simulink library "misc_modbus_genbatt_lib"  (Simulink 8.1)
settings: Solver=ode45  StartTime=0.0  StopTime=10.0  RelTol=1e-3
libraries: rtio_generic_modbus x3, simulink x1
settings Model: Creator=RE25624  LastModifiedBy=RE25624

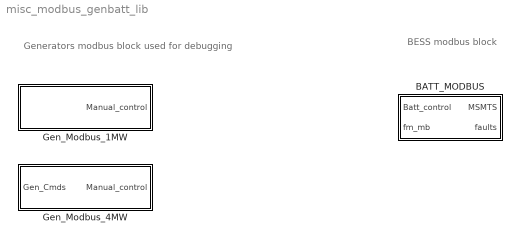
== system misc_modbus_genbatt_lib ==
  note: BESS modbus block
  note: Generators modbus block used for debugging
  BATT_MODBUS : Subsystem
  Gen_Modbus_1MW : Subsystem
  Gen_Modbus_4MW : Subsystem

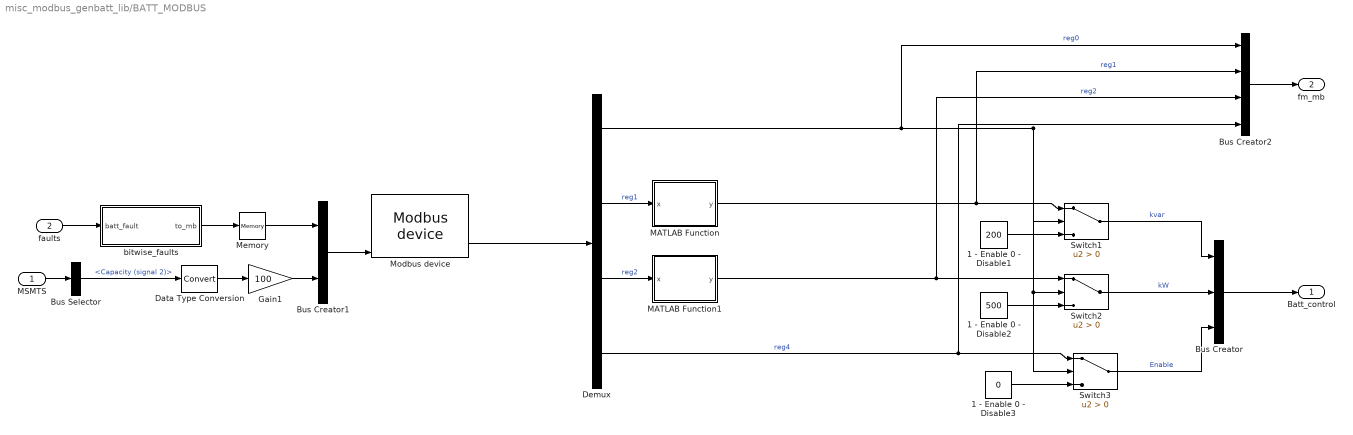
== system misc_modbus_genbatt_lib/BATT_MODBUS ==
  MSMTS : Inport
  faults : Inport  Port=2
  1 - Enable 0 - Disable1 : Constant  Value=200
  1 - Enable 0 - Disable2 : Constant  Value=500
  1 - Enable 0 - Disable3 : Constant  Value=0
  Bus Creator : BusCreator  Inputs=3
  Bus Creator1 : BusCreator  Inputs=2
  Bus Creator2 : BusCreator
  Bus Selector : BusSelector  OutputSignals=Capacity (signal 2)
  Data Type Conversion : DataTypeConversion
  Demux : Demux
  Gain1 : Gain  Gain=100
  MATLAB Function : MATLAB Function  TreatAsAtomicUnit=on
  MATLAB Function1 : MATLAB Function  TreatAsAtomicUnit=on
  Memory : Memory
  Modbus device : rtio_generic_modbus/Modbus device  conf_name=batt_slave_cfg.opal  conf_name_mask=batt_slave_cfg.xls  sample_time=Ts
  Switch1 : Switch  Criteria=u2 > Threshold
  Switch2 : Switch  Criteria=u2 > Threshold
  Switch3 : Switch  Criteria=u2 > Threshold
  bitwise_faults : Subsystem
  Batt_control : Outport
  fm_mb : Outport  Port=2
  wires:
  Modbus device/2 -> Demux/1
  1 - Enable 0 - Disable1/1 -> Switch1/3
  1 - Enable 0 - Disable2/1 -> Switch2/3
  1 - Enable 0 - Disable3/1 -> Switch3/3
  Demux/2 -> MATLAB Function/1(x)  "reg1"
  Demux/3 -> MATLAB Function1/1(x)  "reg2"
  Demux/4 -> Switch3/1, Bus Creator2/4  "reg4"
  Demux/1 -> Switch1/2, Switch2/2, Switch3/2, Bus Creator2/1  "reg0"
  Switch1/1 -> Bus Creator/1  "kvar"
  Switch2/1 -> Bus Creator/2  "kW"
  Switch3/1 -> Bus Creator/3  "Enable"
  Bus Creator/1 -> Batt_control/1
  MSMTS/1 -> Bus Selector/1
  Bus Selector/1 -> Data Type Conversion/1  "<Capacity (signal 2)>"
  Data Type Conversion/1 -> Gain1/1
  Bus Creator1/1 -> Modbus device/4
  Gain1/1 -> Bus Creator1/2
  Bus Creator2/1 -> fm_mb/1
  bitwise_faults/1(to_mb) -> Memory/1
  faults/1 -> bitwise_faults/1(batt_fault)
  Memory/1 -> Bus Creator1/1
  MATLAB Function1/1(y) -> Switch2/1, Bus Creator2/3  "reg2"
  MATLAB Function/1(y) -> Switch1/1, Bus Creator2/2  "reg1"

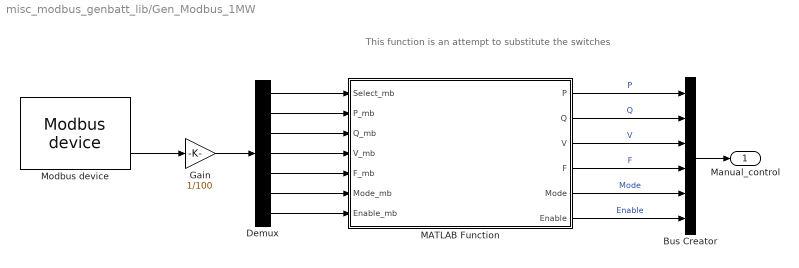
== system misc_modbus_genbatt_lib/Gen_Modbus_1MW ==
  note: This function is an attempt to substitute the switches
  Bus Creator : BusCreator  Inputs=6
  Demux : Demux  Outputs=7
  Gain : Gain  Gain=1/100
  MATLAB Function : MATLAB Function  TreatAsAtomicUnit=on
  Modbus device : rtio_generic_modbus/Modbus device  conf_name=none  conf_name_mask=gen_slave_cfg2.xls  sample_time=Ts
  Manual_control : Outport
  wires:
  MATLAB Function/6(Enable) -> Bus Creator/6  "Enable"
  MATLAB Function/5(Mode) -> Bus Creator/5  "Mode"
  MATLAB Function/4(F) -> Bus Creator/4  "F"
  MATLAB Function/3(V) -> Bus Creator/3  "V"
  MATLAB Function/2(Q) -> Bus Creator/2  "Q"
  MATLAB Function/1(P) -> Bus Creator/1  "P"
  Bus Creator/1 -> Manual_control/1
  Demux/7 -> MATLAB Function/7(Enable_mb)
  Demux/6 -> MATLAB Function/6(Mode_mb)
  Demux/5 -> MATLAB Function/5(F_mb)
  Demux/4 -> MATLAB Function/4(V_mb)
  Demux/3 -> MATLAB Function/3(Q_mb)
  Demux/2 -> MATLAB Function/2(P_mb)
  Demux/1 -> MATLAB Function/1(Select_mb)
  Modbus device/2 -> Gain/1
  Gain/1 -> Demux/1

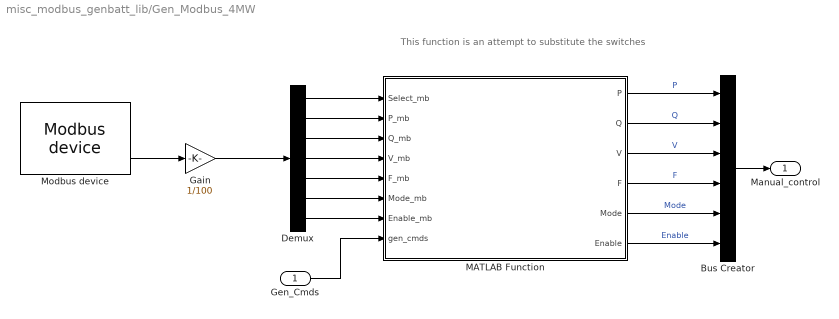
== system misc_modbus_genbatt_lib/Gen_Modbus_4MW ==
  note: This function is an attempt to substitute the switches
  Gen_Cmds : Inport
  Bus Creator : BusCreator  Inputs=6
  Demux : Demux  Outputs=7
  Gain : Gain  Gain=1/100
  MATLAB Function : MATLAB Function  TreatAsAtomicUnit=on
  Modbus device : rtio_generic_modbus/Modbus device  conf_name=gen_slave_cfg.opal  conf_name_mask=gen_slave_cfg.xls  sample_time=Ts
  Manual_control : Outport
  wires:
  Gen_Cmds/1 -> MATLAB Function/8(gen_cmds)
  Modbus device/2 -> Gain/1
  MATLAB Function/6(Enable) -> Bus Creator/6  "Enable"
  MATLAB Function/5(Mode) -> Bus Creator/5  "Mode"
  MATLAB Function/4(F) -> Bus Creator/4  "F"
  MATLAB Function/3(V) -> Bus Creator/3  "V"
  MATLAB Function/2(Q) -> Bus Creator/2  "Q"
  MATLAB Function/1(P) -> Bus Creator/1  "P"
  Bus Creator/1 -> Manual_control/1
  Demux/7 -> MATLAB Function/7(Enable_mb)
  Demux/6 -> MATLAB Function/6(Mode_mb)
  Demux/5 -> MATLAB Function/5(F_mb)
  Demux/4 -> MATLAB Function/4(V_mb)
  Demux/3 -> MATLAB Function/3(Q_mb)
  Demux/2 -> MATLAB Function/2(P_mb)
  Demux/1 -> MATLAB Function/1(Select_mb)
  Gain/1 -> Demux/1

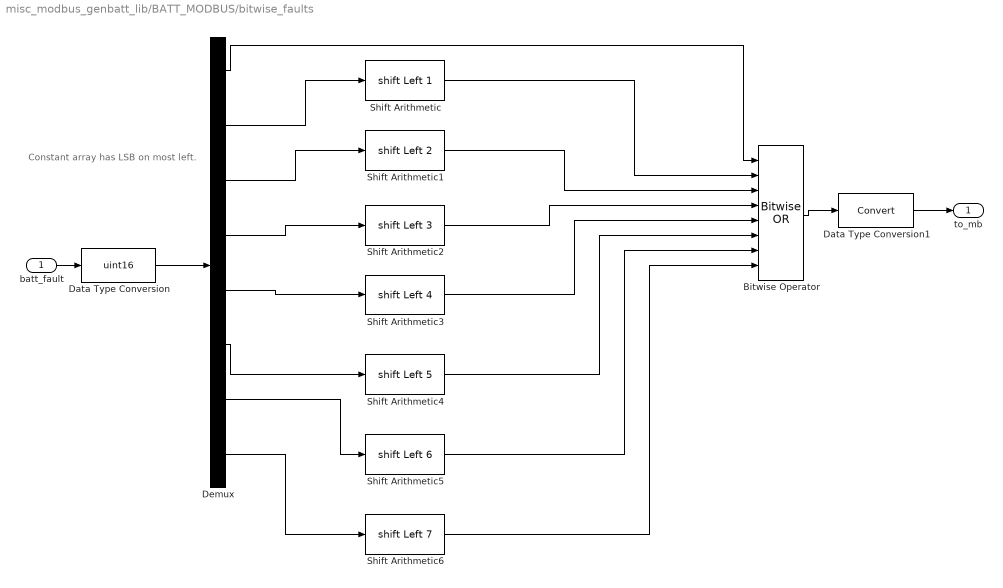
== system misc_modbus_genbatt_lib/BATT_MODBUS/bitwise_faults ==
  note: Constant array has LSB on most left.
  batt_fault : Inport
  Bitwise Operator : simulink/Logic and Bit Operations/Bitwise Operator  logicop=OR  UseBitMask=off  NumInputPorts=8  BitMask=bin2dec('11011001')  BitMaskRealWorld=Stored Integer
  Data Type Conversion : DataTypeConversion  OutDataTypeStr=uint16
  Data Type Conversion1 : DataTypeConversion
  Demux : Demux  Outputs=8
  Shift Arithmetic : ArithShift  BitShiftNumber=1  BitShiftDirection=Left
  Shift Arithmetic1 : ArithShift  BitShiftNumber=2  BitShiftDirection=Left
  Shift Arithmetic2 : ArithShift  BitShiftNumber=3  BitShiftDirection=Left
  Shift Arithmetic3 : ArithShift  BitShiftNumber=4  BitShiftDirection=Left
  Shift Arithmetic4 : ArithShift  BitShiftNumber=5  BitShiftDirection=Left
  Shift Arithmetic5 : ArithShift  BitShiftNumber=6  BitShiftDirection=Left
  Shift Arithmetic6 : ArithShift  BitShiftNumber=7  BitShiftDirection=Left
  to_mb : Outport
  wires:
  Data Type Conversion1/1 -> to_mb/1
  Bitwise Operator/1 -> Data Type Conversion1/1
  batt_fault/1 -> Data Type Conversion/1
  Demux/6 -> Shift Arithmetic4/1
  Demux/5 -> Shift Arithmetic3/1
  Demux/4 -> Shift Arithmetic2/1
  Demux/3 -> Shift Arithmetic1/1
  Demux/2 -> Shift Arithmetic/1
  Demux/1 -> Bitwise Operator/1
  Data Type Conversion/1 -> Demux/1
  Demux/7 -> Shift Arithmetic5/1
  Demux/8 -> Shift Arithmetic6/1
  Shift Arithmetic/1 -> Bitwise Operator/2
  Shift Arithmetic1/1 -> Bitwise Operator/3
  Shift Arithmetic2/1 -> Bitwise Operator/4
  Shift Arithmetic3/1 -> Bitwise Operator/5
  Shift Arithmetic4/1 -> Bitwise Operator/6
  Shift Arithmetic5/1 -> Bitwise Operator/7
  Shift Arithmetic6/1 -> Bitwise Operator/8

== matlab function Gen_Modbus_1MW/MATLAB Function ==
  data: Select_mb input double; P output double; P_mb input double; Q_mb input double; V_mb input double; F_mb input double; Mode_mb input double; Enable_mb input double; Q output double; V output double; F output double; Mode output double; Enable output double
function [P,Q,V,F,Mode,Enable] = genmb_1MW(Select_mb, P_mb, Q_mb, V_mb, F_mb, Mode_mb, Enable_mb)
%#codegen

if Select_mb == 1
    P = P_mb;
    Q = Q_mb;
    V = V_mb;
    F = F_mb;
    Mode = Mode_mb;
    Enable = Enable_mb;
else
    P = 0.8;
    Q = 0.2;
    V = 1;
    F = 1;
    Mode = 1;
    Enable = 1;
end

== matlab function Gen_Modbus_4MW/MATLAB Function ==
  data: Select_mb input double; P output double; P_mb input double; Q_mb input double; V_mb input double; F_mb input double; Mode_mb input double; Enable_mb input double; Q output double; V output double; F output double; Mode output double; Enable output double; gen_cmds input double
function [P,Q,V,F,Mode,Enable] = genmb_4MW(Select_mb, P_mb, Q_mb, V_mb, F_mb, Mode_mb, Enable_mb, gen_cmds)
%#codegen

% gen_cmds mapping
if isempty(gen_cmds)
    Sync = 0;
    V_sync = 0;
    F_sync = 0;
    Mode_sync = 0;
else
    V_sync = gen_cmds(1);
    F_sync = gen_cmds(2);
    Mode_sync = gen_cmds(3);
    Sync = gen_cmds(4);
end

if Sync == 1
    VFM_select = 2;
else
    VFM_select = Select_mb;
end

if VFM_select == 1
    P = P_mb;
    Q = Q_mb;
    V = V_mb;
    F = F_mb;
    Mode = Mode_mb;
    Enable = Enable_mb;
elseif VFM_select == 2
    P = P_mb;
    Q = Q_mb;
    V = V_sync; % sync parameters
    F = F_sync;
    Mode = Mode_sync;
    Enable = Enable_mb;
else
    P = 0.8;
    Q = 0.2;
    V = 1;
    F = 1;
    Mode = 1;
    Enable = 1;
end

== matlab function BATT_MODBUS/MATLAB Function ==
  data: x input double; y output double
function y = fcn(x)
%#codegen

r=typecast(uint16(x),'int16');
y=double(r(1));

== matlab function BATT_MODBUS/MATLAB Function1 ==
  data: x input double; y output double
function y = fcn(x)
%#codegen

r=typecast(uint16(x),'int16');
y=double(r(1));
